simulink model "shiftregister1"  (R2023a)
settings: Solver=VariableStepAuto  StartTime=0.0  StopTime=10.0  RelTol=1e-3
libraries: NSA_DEVS_SINKS x6, NSA_DEVS_DIGITAL x5, NSA_DEVS_SOURCES x2, NSA_DEVS_LOGISTICS x2
settings Model: Creator=peter  LastModifiedBy=david

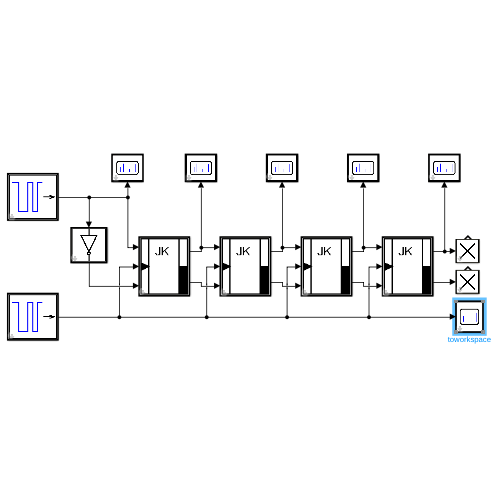
[thumbnail: Simulink's stored preview of the top-level diagram]
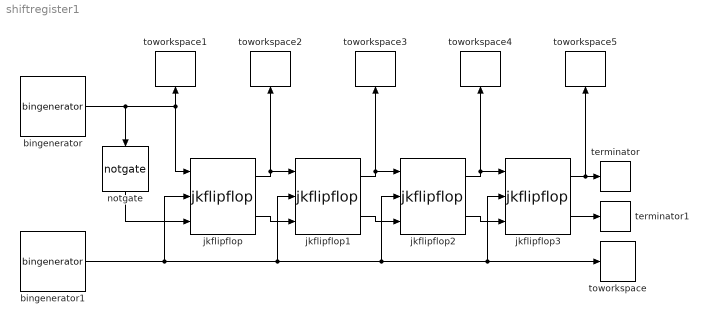
== system shiftregister1 ==
  bingenerator : NSA_DEVS_SOURCES/bingenerator  z0=0  tVec=[1, 2, 3, 4, 7, 9, 100]  tau=[0,1]  debug=0
  bingenerator1 : NSA_DEVS_SOURCES/bingenerator  z0=1  tVec=[0.5, 1.0]  tau=[0,1]  debug=0
  jkflipflop{,1..3} (4 alike) : NSA_DEVS_DIGITAL/jkflipflop  q0=0  tau=[0,1]  debug=0
      settings: LibrarySourceBlock=NSA_DEVS_DIGITAL_FLIPFLOP/jkflipflop
  notgate : NSA_DEVS_DIGITAL/notgate  tau=[0,1]  debug=0
      settings: LibrarySourceBlock=NSA_DEVS_DIGITAL_LOGIC/notgate
  terminator : NSA_DEVS_LOGISTICS/terminator  tau=[0,1]  debug=0
  terminator1 : NSA_DEVS_LOGISTICS/terminator  tau=[0,1]  debug=0
  toworkspace : NSA_DEVS_SINKS/toworkspace  varname="\"bin2Out\""  t0=0  format="\"vector\""  tau=[0,5]  debug=0
  toworkspace1 : NSA_DEVS_SINKS/toworkspace  varname="\"bin1Out\""  t0=0  format="\"vector\""  tau=[0,5]  debug=0
  toworkspace2 : NSA_DEVS_SINKS/toworkspace  varname="\"q1Out\""  t0=0  format="\"vector\""  tau=[0,5]  debug=0
  toworkspace3 : NSA_DEVS_SINKS/toworkspace  varname="\"q2Out\""  t0=0  format="\"vector\""  tau=[0,5]  debug=0
  toworkspace4 : NSA_DEVS_SINKS/toworkspace  varname="\"q3Out\""  t0=0  format="\"vector\""  tau=[0,5]  debug=0
  toworkspace5 : NSA_DEVS_SINKS/toworkspace  varname="\"q4Out\""  t0=0  format="\"vector\""  tau=[0,5]  debug=0
  wires:
  jkflipflop/1 -> toworkspace2/1, jkflipflop1/1
  jkflipflop/2 -> jkflipflop1/3
  jkflipflop1/1 -> toworkspace3/1, jkflipflop2/1
  jkflipflop1/2 -> jkflipflop2/3
  jkflipflop2/1 -> jkflipflop3/1, toworkspace4/1
  jkflipflop2/2 -> jkflipflop3/3
  jkflipflop3/1 -> toworkspace5/1, terminator/1
  jkflipflop3/2 -> terminator1/1
  bingenerator/1 -> notgate/1, jkflipflop/1, toworkspace1/1
  notgate/1 -> jkflipflop/3
  bingenerator1/1 -> jkflipflop/2, jkflipflop1/2, jkflipflop2/2, toworkspace/1, jkflipflop3/2
